simulink model "RocketStability_InitialConditions"  (R2014a)
settings: Solver=ode3  StartTime=0.0  StopTime=25  FixedStep=0.01  MinStep=0.01  RelTol=1e-3
libraries: rocket_vertical_flight_library x1, rocket_angular_flight_library x1
settings Model: Creator=scorpii  LastModifiedBy=scorpii
settings SolverCC: InitialStep=0.01
settings DataIOCC: LimitDataPoints=off
settings OptimizationCC: SimCompilerOptimization=off
settings DebuggingCC: ArtificialAlgebraicLoopMsg=error  MergeDetectMultiDrivingBlocksExec=error  FrameProcessingCompatibilityMsg=error
settings RTWCC: RTWCompilerOptimization=off

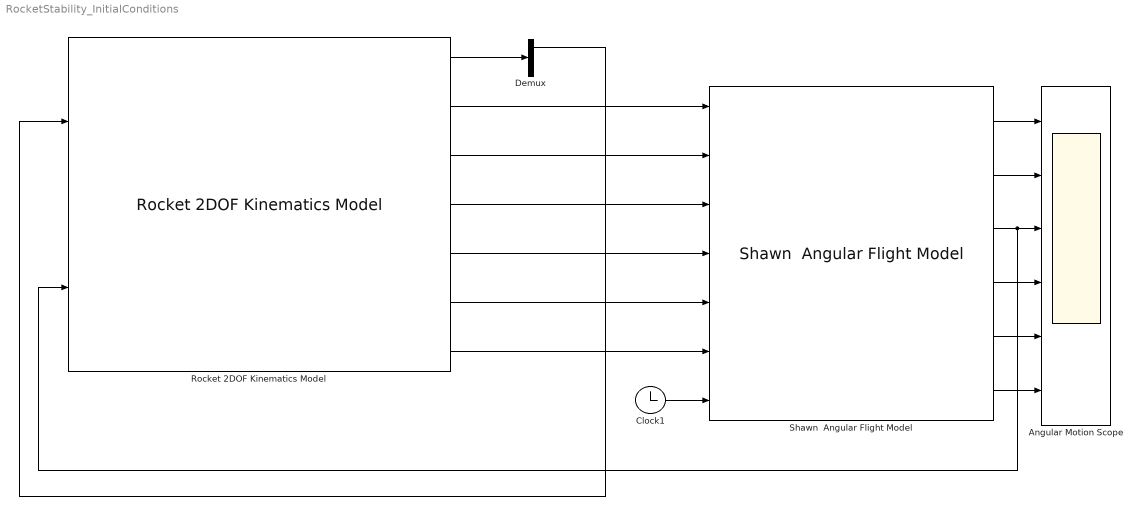
== system RocketStability_InitialConditions ==
  Angular Motion Scope : Scope  NumInputPorts=6
      settings: TimeRange=10  YMin=-0.7~-0.125~-0.015~0.05~9~-5  YMax=0.9~0.125~0.015~0.275~24~5  SaveName=ScopeData5
  Clock1 : Clock
  Demux : Demux  Outputs=2
  Rocket 2DOF Kinematics Model : rocket_vertical_flight_library/Rocket 2DOF Kinematics Model
  Shawn  Angular Flight Model : rocket_angular_flight_library/Shawn  Angular Flight Model
  wires:
  Shawn  Angular Flight Model/2 -> Angular Motion Scope/2
  Shawn  Angular Flight Model/1 -> Angular Motion Scope/1
  Clock1/1 -> Shawn  Angular Flight Model/7
  Shawn  Angular Flight Model/5 -> Angular Motion Scope/5
  Shawn  Angular Flight Model/4 -> Angular Motion Scope/4
  Shawn  Angular Flight Model/6 -> Angular Motion Scope/6
  Shawn  Angular Flight Model/3 -> Rocket 2DOF Kinematics Model/2, Angular Motion Scope/3
  Demux/1 -> Rocket 2DOF Kinematics Model/1
  Rocket 2DOF Kinematics Model/1 -> Demux/1
  Rocket 2DOF Kinematics Model/2 -> Shawn  Angular Flight Model/1
  Rocket 2DOF Kinematics Model/3 -> Shawn  Angular Flight Model/2
  Rocket 2DOF Kinematics Model/4 -> Shawn  Angular Flight Model/3
  Rocket 2DOF Kinematics Model/5 -> Shawn  Angular Flight Model/4
  Rocket 2DOF Kinematics Model/6 -> Shawn  Angular Flight Model/5
  Rocket 2DOF Kinematics Model/7 -> Shawn  Angular Flight Model/6
